simulink model "Switching_06"  (R2022b)
settings: Solver=ode4  StartTime=0.0  StopTime=50  FixedStep=1e-3  MaxStep=1e-3  RelTol=1e-3
undefined symbols (not defined in the file or in its folder): p1, p2, p3, PR_k1, PR_k2, PR_k3, SF_b, SF_xi1, theta_d, tolerance_posture, v_sat, w_sat, x_d, y_d
libraries: simulink x18, dspsigops x6
settings Model: Creator=david  LastModifiedBy=david

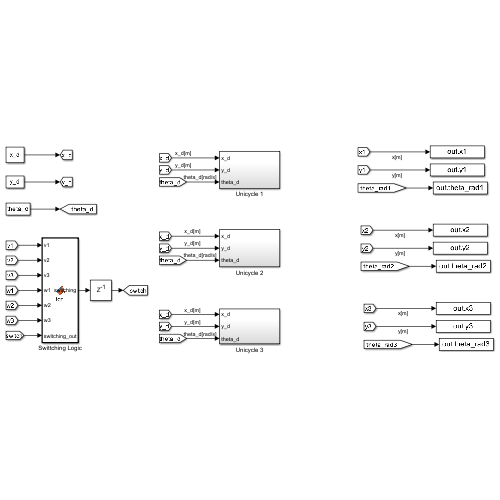
[thumbnail: Simulink's stored preview of the top-level diagram]
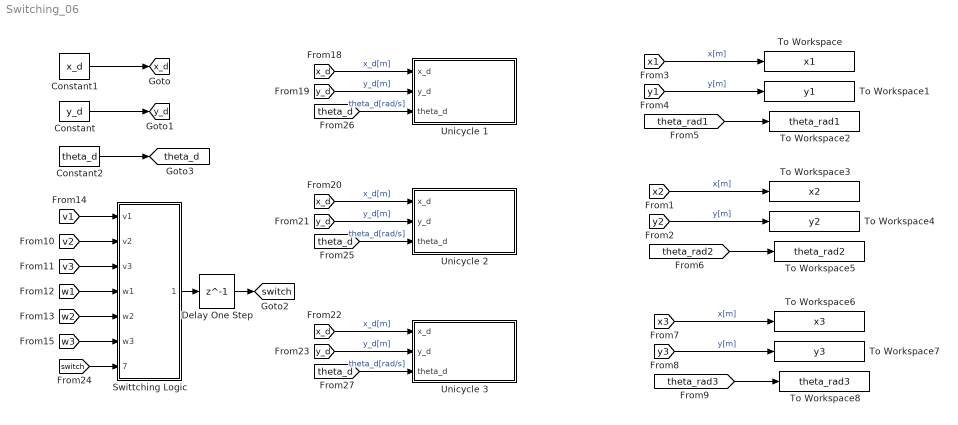
== system Switching_06 ==
  Constant : Constant  Value=y_d
  Constant1 : Constant  Value=x_d
  Constant2 : Constant  Value=theta_d
  Delay One Step : Delay  DelayLength=1
  Swittching Logic : MATLAB Function  TreatAsAtomicUnit=on
  To Workspace : ToWorkspace  VariableName=x1  SaveFormat=Structure With Time  SampleTime=-1
  To Workspace1 : ToWorkspace  VariableName=y1  SaveFormat=Structure With Time  SampleTime=-1
  To Workspace2 : ToWorkspace  VariableName=theta_rad1  SaveFormat=Structure With Time  SampleTime=-1
  To Workspace3 : ToWorkspace  VariableName=x2  SaveFormat=Structure With Time  SampleTime=-1
  To Workspace4 : ToWorkspace  VariableName=y2  SaveFormat=Structure With Time  SampleTime=-1
  To Workspace5 : ToWorkspace  VariableName=theta_rad2  SaveFormat=Structure With Time  SampleTime=-1
  To Workspace6 : ToWorkspace  VariableName=x3  SaveFormat=Structure With Time  SampleTime=-1
  To Workspace7 : ToWorkspace  VariableName=y3  SaveFormat=Structure With Time  SampleTime=-1
  To Workspace8 : ToWorkspace  VariableName=theta_rad3  SaveFormat=Structure With Time  SampleTime=-1
  Unicycle 1 : Subsystem
  Unicycle 2 : Subsystem
  Unicycle 3 : Subsystem
  tag scope: switch=global, theta_d=global, x_d=global, y_d=global
  wires:
  [x1] -> To Workspace/1  "x[m]"
  [y1] -> To Workspace1/1  "y[m]"
  [theta_rad1] -> To Workspace2/1
  [x2] -> To Workspace3/1  "x[m]"
  [y2] -> To Workspace4/1  "y[m]"
  [theta_rad2] -> To Workspace5/1
  [theta_rad3] -> To Workspace8/1
  [y3] -> To Workspace7/1  "y[m]"
  [x3] -> To Workspace6/1  "x[m]"
  [w2] -> Swittching Logic/5(w2)
  [v1] -> Swittching Logic/1(v1)
  [v2] -> Swittching Logic/2(v2)
  Constant2/1 -> [theta_d]
  [w1] -> Swittching Logic/4(w1)
  [v3] -> Swittching Logic/3(v3)
  [x_d] -> Unicycle 1/1(x_d)  "x_d[m]"
  [y_d] -> Unicycle 3/2(y_d)  "y_d[m]"
  [switch] -> Swittching Logic/7(switching_out)
  Swittching Logic/1(switching) -> Delay One Step/1
  [theta_d] -> Unicycle 3/3(theta_d)  "theta_d[rad/s]"
  [x_d] -> Unicycle 2/1(x_d)  "x_d[m]"
  [w3] -> Swittching Logic/6(w3)
  Constant/1 -> [y_d]
  Delay One Step/1 -> [switch]
  [y_d] -> Unicycle 1/2(y_d)  "y_d[m]"
  [theta_d] -> Unicycle 2/3(theta_d)  "theta_d[rad/s]"
  [y_d] -> Unicycle 2/2(y_d)  "y_d[m]"
  [x_d] -> Unicycle 3/1(x_d)  "x_d[m]"
  Constant1/1 -> [x_d]
  [theta_d] -> Unicycle 1/3(theta_d)  "theta_d[rad/s]"

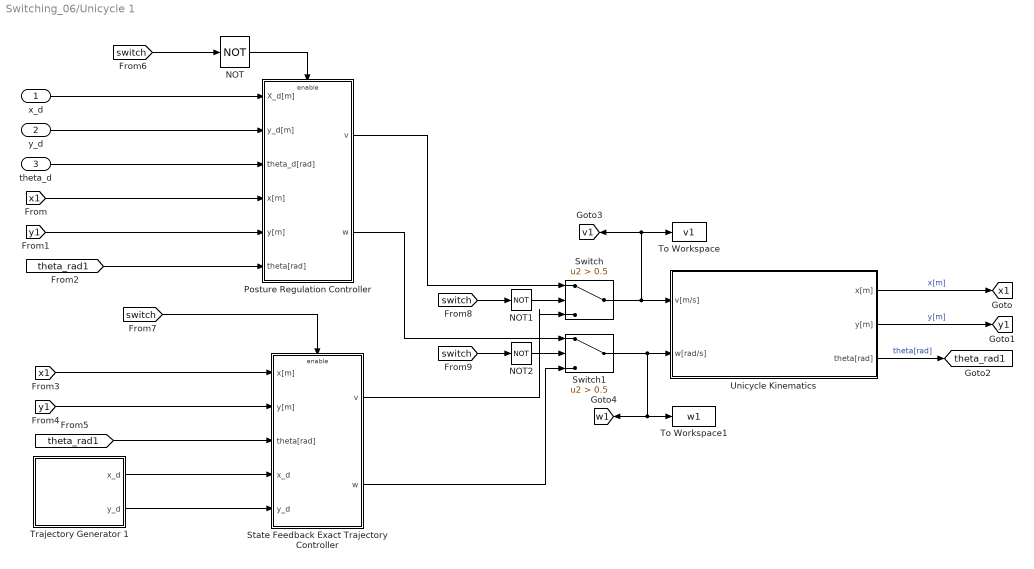
== system Switching_06/Unicycle 1 ==
  x_d : Inport
  y_d : Inport  Port=2
  theta_d : Inport  Port=3
  NOT : Logic  Operator=NOT  IconShape=distinctive  AllPortsSameDT=off  OutDataTypeStr=boolean
  NOT1 : Logic  Operator=NOT  IconShape=distinctive  AllPortsSameDT=off  OutDataTypeStr=boolean
  NOT2 : Logic  Operator=NOT  IconShape=distinctive  AllPortsSameDT=off  OutDataTypeStr=boolean
  Posture Regulation Controller : Subsystem
  State Feedback Exact Trajectory Controller : Subsystem
  Switch : Switch  Criteria=u2 > Threshold  Threshold=0.5  SaturateOnIntegerOverflow=off  InputSameDT=off
  Switch1 : Switch  Criteria=u2 > Threshold  Threshold=0.5  SaturateOnIntegerOverflow=off  InputSameDT=off
  To Workspace : ToWorkspace  VariableName=v1  SaveFormat=Structure With Time  SampleTime=-1
  To Workspace1 : ToWorkspace  VariableName=w1  SaveFormat=Structure With Time  SampleTime=-1
  "Trajectory Generator 1 " : Subsystem
  Unicycle Kinematics : Subsystem
  tag scope: theta_rad1=global, v1=global, w1=global, x1=global, y1=global
  wires:
  Unicycle Kinematics/3(theta[rad]) -> [theta_rad1]  "theta[rad]"
  Unicycle Kinematics/2(y[m]) -> [y1]  "y[m]"
  Unicycle Kinematics/1(x[m]) -> [x1]  "x[m]"
  [theta_rad1] -> State Feedback Exact Trajectory Controller/3(theta[rad])
  [x1] -> State Feedback Exact Trajectory Controller/1(x[m])
  [y1] -> State Feedback Exact Trajectory Controller/2(y[m])
  "Trajectory Generator 1 "/1(x_d) -> State Feedback Exact Trajectory Controller/4(x_d)
  "Trajectory Generator 1 "/2(y_d) -> State Feedback Exact Trajectory Controller/5(y_d)
  [switch] -> State Feedback Exact Trajectory Controller/Enable
  Posture Regulation Controller/2(w) -> Switch1/1
  Posture Regulation Controller/1(v) -> Switch/1
  State Feedback Exact Trajectory Controller/2(w) -> Switch1/3
  [switch] -> NOT2/1
  State Feedback Exact Trajectory Controller/1(v) -> Switch/3
  [switch] -> NOT1/1
  NOT1/1 -> Switch/2
  NOT2/1 -> Switch1/2
  Switch/1 -> Unicycle Kinematics/1(v[m/s]), [v1], To Workspace/1
  Switch1/1 -> Unicycle Kinematics/2(w[rad/s]), To Workspace1/1, [w1]
  [x1] -> Posture Regulation Controller/4(x[m])
  [switch] -> NOT/1
  x_d/1 -> Posture Regulation Controller/1(X_d[m])
  [theta_rad1] -> Posture Regulation Controller/6(theta[rad])
  [y1] -> Posture Regulation Controller/5(y[m])
  y_d/1 -> Posture Regulation Controller/2(y_d[m])
  NOT/1 -> Posture Regulation Controller/Enable
  theta_d/1 -> Posture Regulation Controller/3(theta_d[rad])

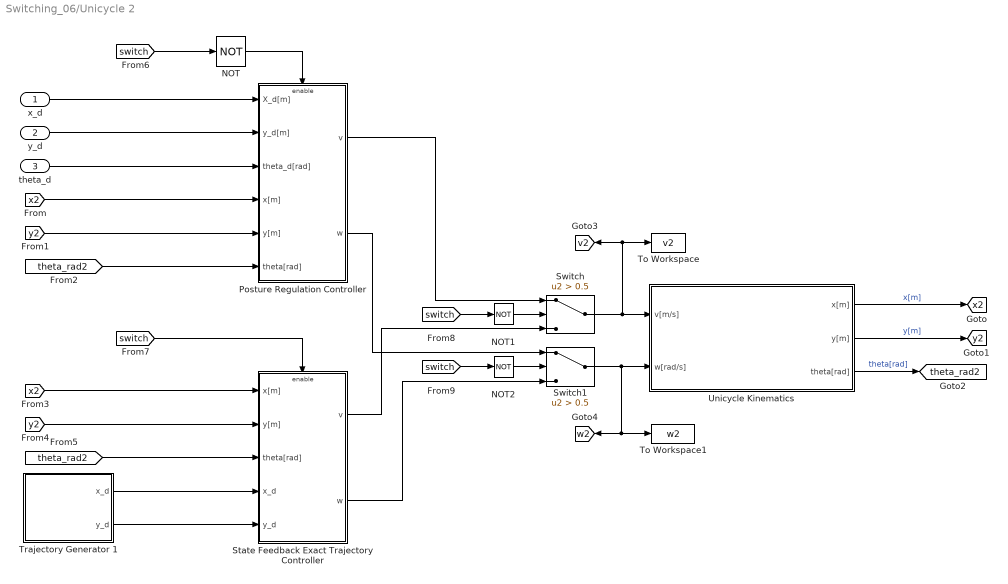
== system Switching_06/Unicycle 2 ==
  x_d : Inport
  y_d : Inport  Port=2
  theta_d : Inport  Port=3
  NOT : Logic  Operator=NOT  IconShape=distinctive  AllPortsSameDT=off  OutDataTypeStr=boolean
  NOT1 : Logic  Operator=NOT  IconShape=distinctive  AllPortsSameDT=off  OutDataTypeStr=boolean
  NOT2 : Logic  Operator=NOT  IconShape=distinctive  AllPortsSameDT=off  OutDataTypeStr=boolean
  Posture Regulation Controller : Subsystem
  State Feedback Exact Trajectory Controller : Subsystem
  Switch : Switch  Criteria=u2 > Threshold  Threshold=0.5  SaturateOnIntegerOverflow=off  InputSameDT=off
  Switch1 : Switch  Criteria=u2 > Threshold  Threshold=0.5  SaturateOnIntegerOverflow=off  InputSameDT=off
  To Workspace : ToWorkspace  VariableName=v2  SaveFormat=Structure With Time  SampleTime=-1
  To Workspace1 : ToWorkspace  VariableName=w2  SaveFormat=Structure With Time  SampleTime=-1
  "Trajectory Generator 1 " : Subsystem
  Unicycle Kinematics : Subsystem
  tag scope: theta_rad2=global, v2=global, w2=global, x2=global, y2=global
  wires:
  Unicycle Kinematics/3(theta[rad]) -> [theta_rad2]  "theta[rad]"
  Unicycle Kinematics/2(y[m]) -> [y2]  "y[m]"
  Unicycle Kinematics/1(x[m]) -> [x2]  "x[m]"
  [switch] -> State Feedback Exact Trajectory Controller/Enable
  Posture Regulation Controller/2(w) -> Switch1/1
  Posture Regulation Controller/1(v) -> Switch/1
  State Feedback Exact Trajectory Controller/2(w) -> Switch1/3
  [switch] -> NOT2/1
  Switch1/1 -> [w2], To Workspace1/1, Unicycle Kinematics/2(w[rad/s])
  [switch] -> NOT1/1
  NOT1/1 -> Switch/2
  NOT2/1 -> Switch1/2
  State Feedback Exact Trajectory Controller/1(v) -> Switch/3
  [theta_rad2] -> State Feedback Exact Trajectory Controller/3(theta[rad])
  [x2] -> State Feedback Exact Trajectory Controller/1(x[m])
  [y2] -> State Feedback Exact Trajectory Controller/2(y[m])
  "Trajectory Generator 1 "/1(x_d) -> State Feedback Exact Trajectory Controller/4(x_d)
  "Trajectory Generator 1 "/2(y_d) -> State Feedback Exact Trajectory Controller/5(y_d)
  theta_d/1 -> Posture Regulation Controller/3(theta_d[rad])
  x_d/1 -> Posture Regulation Controller/1(X_d[m])
  [switch] -> NOT/1
  [x2] -> Posture Regulation Controller/4(x[m])
  [y2] -> Posture Regulation Controller/5(y[m])
  NOT/1 -> Posture Regulation Controller/Enable
  y_d/1 -> Posture Regulation Controller/2(y_d[m])
  [theta_rad2] -> Posture Regulation Controller/6(theta[rad])
  Switch/1 -> To Workspace/1, [v2], Unicycle Kinematics/1(v[m/s])

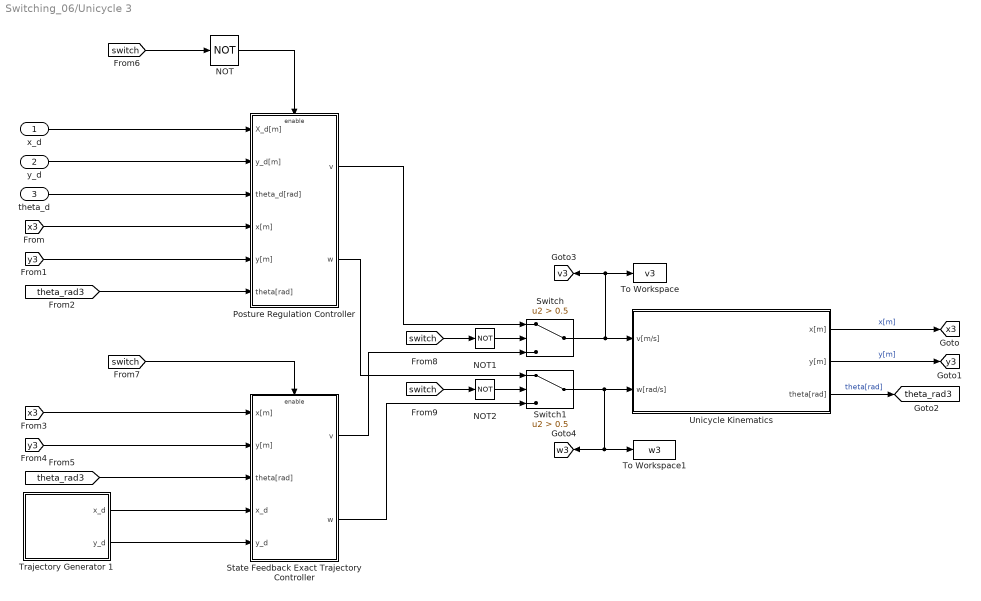
== system Switching_06/Unicycle 3 ==
  x_d : Inport
  y_d : Inport  Port=2
  theta_d : Inport  Port=3
  NOT : Logic  Operator=NOT  IconShape=distinctive  AllPortsSameDT=off  OutDataTypeStr=boolean
  NOT1 : Logic  Operator=NOT  IconShape=distinctive  AllPortsSameDT=off  OutDataTypeStr=boolean
  NOT2 : Logic  Operator=NOT  IconShape=distinctive  AllPortsSameDT=off  OutDataTypeStr=boolean
  Posture Regulation Controller : Subsystem
  State Feedback Exact Trajectory Controller : Subsystem
  Switch : Switch  Criteria=u2 > Threshold  Threshold=0.5  SaturateOnIntegerOverflow=off  InputSameDT=off
  Switch1 : Switch  Criteria=u2 > Threshold  Threshold=0.5  SaturateOnIntegerOverflow=off  InputSameDT=off
  To Workspace : ToWorkspace  VariableName=v3  SaveFormat=Structure With Time  SampleTime=-1
  To Workspace1 : ToWorkspace  VariableName=w3  SaveFormat=Structure With Time  SampleTime=-1
  "Trajectory Generator 1 " : Subsystem
  Unicycle Kinematics : Subsystem
  tag scope: theta_rad3=global, v3=global, w3=global, x3=global, y3=global
  wires:
  Unicycle Kinematics/3(theta[rad]) -> [theta_rad3]  "theta[rad]"
  Unicycle Kinematics/2(y[m]) -> [y3]  "y[m]"
  Unicycle Kinematics/1(x[m]) -> [x3]  "x[m]"
  [switch] -> State Feedback Exact Trajectory Controller/Enable
  Posture Regulation Controller/1(v) -> Switch/1
  [switch] -> NOT1/1
  [switch] -> NOT2/1
  Posture Regulation Controller/2(w) -> Switch1/1
  NOT1/1 -> Switch/2
  NOT2/1 -> Switch1/2
  [theta_rad3] -> State Feedback Exact Trajectory Controller/3(theta[rad])
  [x3] -> State Feedback Exact Trajectory Controller/1(x[m])
  [y3] -> State Feedback Exact Trajectory Controller/2(y[m])
  "Trajectory Generator 1 "/1(x_d) -> State Feedback Exact Trajectory Controller/4(x_d)
  "Trajectory Generator 1 "/2(y_d) -> State Feedback Exact Trajectory Controller/5(y_d)
  State Feedback Exact Trajectory Controller/1(v) -> Switch/3
  State Feedback Exact Trajectory Controller/2(w) -> Switch1/3
  Switch/1 -> Unicycle Kinematics/1(v[m/s]), To Workspace/1, [v3]
  Switch1/1 -> [w3], To Workspace1/1, Unicycle Kinematics/2(w[rad/s])
  y_d/1 -> Posture Regulation Controller/2(y_d[m])
  [y3] -> Posture Regulation Controller/5(y[m])
  [x3] -> Posture Regulation Controller/4(x[m])
  x_d/1 -> Posture Regulation Controller/1(X_d[m])
  theta_d/1 -> Posture Regulation Controller/3(theta_d[rad])
  [switch] -> NOT/1
  NOT/1 -> Posture Regulation Controller/Enable
  [theta_rad3] -> Posture Regulation Controller/6(theta[rad])

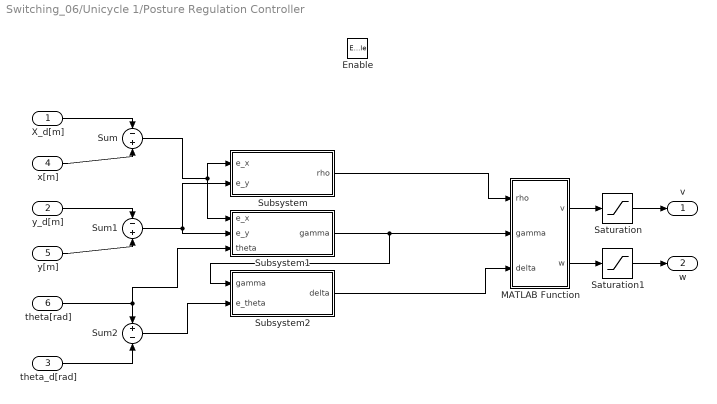
== system Switching_06/Unicycle 1/Posture Regulation Controller ==
  X_d[m] : Inport
  y_d[m] : Inport  Port=2
  theta_d[rad] : Inport  Port=3
  x[m] : Inport  Port=4
  y[m] : Inport  Port=5
  theta[rad] : Inport  Port=6
  Enable : EnablePort
  MATLAB Function : MATLAB Function  TreatAsAtomicUnit=on
  Saturation : Saturate  UpperLimit=v_sat  LowerLimit=-v_sat
  Saturation1 : Saturate  UpperLimit=w_sat  LowerLimit=-w_sat
  Subsystem : Subsystem
  Subsystem1 : Subsystem
  Subsystem2 : Subsystem
  Sum : Sum  Inputs=-+
  Sum1 : Sum  Inputs=-+
  Sum2 : Sum  Inputs=+-
  v : Outport
  w : Outport  Port=2
  wires:
  X_d[m]/1 -> Sum/1
  x[m]/1 -> Sum/2
  y_d[m]/1 -> Sum1/1
  y[m]/1 -> Sum1/2
  Sum1/1 -> Subsystem1/2(e_y), Subsystem/2(e_y)
  Sum2/1 -> Subsystem2/2(e_theta)
  Subsystem1/1(gamma) -> MATLAB Function/2(gamma), Subsystem2/1(gamma)
  Subsystem2/1(delta) -> MATLAB Function/3(delta)
  Subsystem/1(rho) -> MATLAB Function/1(rho)
  Sum/1 -> Subsystem1/1(e_x), Subsystem/1(e_x)
  MATLAB Function/1(v) -> Saturation/1
  MATLAB Function/2(w) -> Saturation1/1
  theta[rad]/1 -> Sum2/1, Subsystem1/3(theta)
  theta_d[rad]/1 -> Sum2/2
  Saturation/1 -> v/1
  Saturation1/1 -> w/1

== system Switching_06/Unicycle 1/State Feedback Exact Trajectory Controller ==
  x[m] : Inport
  y[m] : Inport  Port=2
  theta[rad] : Inport  Port=3
  x_d : Inport  Port=4
  y_d : Inport  Port=5
  Enable : EnablePort
  Controller : Subsystem
  Differential Flatness : Subsystem
  v : Outport
  w : Outport  Port=2
  wires:
  Controller/2(w) -> w/1
  Controller/1(v) -> v/1
  Differential Flatness/3(w_d) -> Controller/3(w_d)
  Differential Flatness/1(q_d) -> Controller/1(q_d)
  Differential Flatness/2(v_d) -> Controller/2(v_d)
  y_d/1 -> Differential Flatness/2(y_d)
  x_d/1 -> Differential Flatness/1(x_d)
  x[m]/1 -> Controller/4(x)
  y[m]/1 -> Controller/5(y)
  theta[rad]/1 -> Controller/6(theta)

== system Switching_06/Unicycle 1/Trajectory Generator 1  ==
  Repeating Sequence : simulink/Sources/Repeating Sequence  rep_seq_t=time  rep_seq_y=y_d1
  Repeating Sequence1 : simulink/Sources/Repeating Sequence  rep_seq_t=time  rep_seq_y=x_d1
  To Workspace2 : ToWorkspace  VariableName=y_d1  SaveFormat=Structure With Time  SampleTime=-1
  To Workspace3 : ToWorkspace  VariableName=x_d1  SaveFormat=Structure With Time  SampleTime=-1
  x_d : Outport
  y_d : Outport  Port=2
  wires:
  Repeating Sequence1/1 -> x_d/1, To Workspace3/1
  Repeating Sequence/1 -> To Workspace2/1, y_d/1

== system Switching_06/Unicycle 1/Unicycle Kinematics ==
  v[m/s] : Inport
  w[rad/s] : Inport  Port=2
  Cos : Trigonometry  Operator=cos
  Cos1 : Trigonometry
  Integrator : Integrator  InitialCondition=p1(1)
  Integrator1 : Integrator  InitialCondition=p1(2)
  Integrator2 : Integrator  InitialCondition=p1(3)
  Product : Product
  Product1 : Product
  x[m] : Outport
  y[m] : Outport  Port=2
  theta[rad] : Outport  Port=3
  wires:
  Integrator/1 -> x[m]/1  "x"
  Integrator1/1 -> y[m]/1  "y"
  w[rad/s]/1 -> Integrator2/1  "theta_dot"
  Integrator2/1 -> Cos/1, Cos1/1, theta[rad]/1  "theta[rad]"
  Product/1 -> Integrator/1  "x_dot"
  Cos1/1 -> Product1/2
  Cos/1 -> Product/1
  v[m/s]/1 -> Product1/1, Product/2
  Product1/1 -> Integrator1/1  "y_dot"

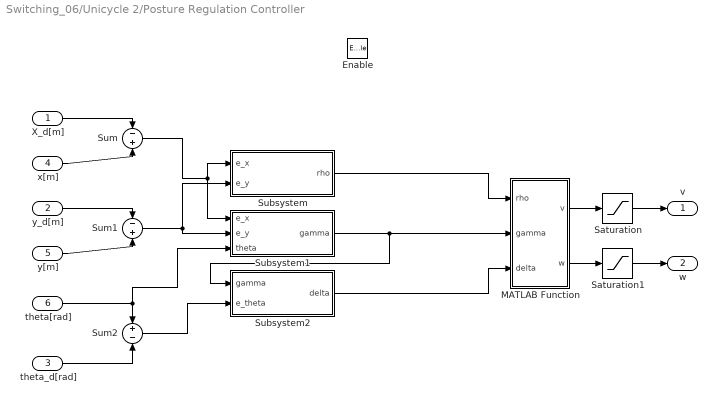
== system Switching_06/Unicycle 2/Posture Regulation Controller ==
  X_d[m] : Inport
  y_d[m] : Inport  Port=2
  theta_d[rad] : Inport  Port=3
  x[m] : Inport  Port=4
  y[m] : Inport  Port=5
  theta[rad] : Inport  Port=6
  Enable : EnablePort
  MATLAB Function : MATLAB Function  TreatAsAtomicUnit=on
  Saturation : Saturate  UpperLimit=v_sat  LowerLimit=-v_sat
  Saturation1 : Saturate  UpperLimit=w_sat  LowerLimit=-w_sat
  Subsystem : Subsystem
  Subsystem1 : Subsystem
  Subsystem2 : Subsystem
  Sum : Sum  Inputs=-+
  Sum1 : Sum  Inputs=-+
  Sum2 : Sum  Inputs=+-
  v : Outport
  w : Outport  Port=2
  wires:
  X_d[m]/1 -> Sum/1
  x[m]/1 -> Sum/2
  y_d[m]/1 -> Sum1/1
  y[m]/1 -> Sum1/2
  Sum1/1 -> Subsystem1/2(e_y), Subsystem/2(e_y)
  Sum2/1 -> Subsystem2/2(e_theta)
  Subsystem1/1(gamma) -> MATLAB Function/2(gamma), Subsystem2/1(gamma)
  Subsystem2/1(delta) -> MATLAB Function/3(delta)
  Subsystem/1(rho) -> MATLAB Function/1(rho)
  Sum/1 -> Subsystem1/1(e_x), Subsystem/1(e_x)
  MATLAB Function/1(v) -> Saturation/1
  MATLAB Function/2(w) -> Saturation1/1
  theta[rad]/1 -> Sum2/1, Subsystem1/3(theta)
  theta_d[rad]/1 -> Sum2/2
  Saturation/1 -> v/1
  Saturation1/1 -> w/1

== system Switching_06/Unicycle 2/State Feedback Exact Trajectory Controller ==
  x[m] : Inport
  y[m] : Inport  Port=2
  theta[rad] : Inport  Port=3
  x_d : Inport  Port=4
  y_d : Inport  Port=5
  Enable : EnablePort
  Controller : Subsystem
  Differential Flatness : Subsystem
  v : Outport
  w : Outport  Port=2
  wires:
  Controller/2(w) -> w/1
  Controller/1(v) -> v/1
  Differential Flatness/3(w_d) -> Controller/3(w_d)
  Differential Flatness/1(q_d) -> Controller/1(q_d)
  Differential Flatness/2(v_d) -> Controller/2(v_d)
  y_d/1 -> Differential Flatness/2(y_d)
  x_d/1 -> Differential Flatness/1(x_d)
  x[m]/1 -> Controller/4(x)
  y[m]/1 -> Controller/5(y)
  theta[rad]/1 -> Controller/6(theta)

== system Switching_06/Unicycle 2/Trajectory Generator 1  ==
  Repeating Sequence : simulink/Sources/Repeating Sequence  rep_seq_t=time  rep_seq_y=y_d2
  Repeating Sequence1 : simulink/Sources/Repeating Sequence  rep_seq_t=time  rep_seq_y=x_d2
  To Workspace2 : ToWorkspace  VariableName=y_d2  SaveFormat=Structure With Time  SampleTime=-1
  To Workspace3 : ToWorkspace  VariableName=x_d2  SaveFormat=Structure With Time  SampleTime=-1
  x_d : Outport
  y_d : Outport  Port=2
  wires:
  Repeating Sequence1/1 -> x_d/1, To Workspace3/1
  Repeating Sequence/1 -> To Workspace2/1, y_d/1

== system Switching_06/Unicycle 2/Unicycle Kinematics ==
  v[m/s] : Inport
  w[rad/s] : Inport  Port=2
  Cos : Trigonometry  Operator=cos
  Cos1 : Trigonometry
  Integrator : Integrator  InitialCondition=p2(1)
  Integrator1 : Integrator  InitialCondition=p2(2)
  Integrator2 : Integrator  InitialCondition=p2(3)
  Product : Product
  Product1 : Product
  x[m] : Outport
  y[m] : Outport  Port=2
  theta[rad] : Outport  Port=3
  wires:
  Integrator/1 -> x[m]/1  "x"
  Integrator1/1 -> y[m]/1  "y"
  w[rad/s]/1 -> Integrator2/1  "theta_dot"
  Integrator2/1 -> Cos/1, Cos1/1, theta[rad]/1  "theta[rad]"
  Product/1 -> Integrator/1  "x_dot"
  Cos1/1 -> Product1/2
  Cos/1 -> Product/1
  v[m/s]/1 -> Product1/1, Product/2
  Product1/1 -> Integrator1/1  "y_dot"

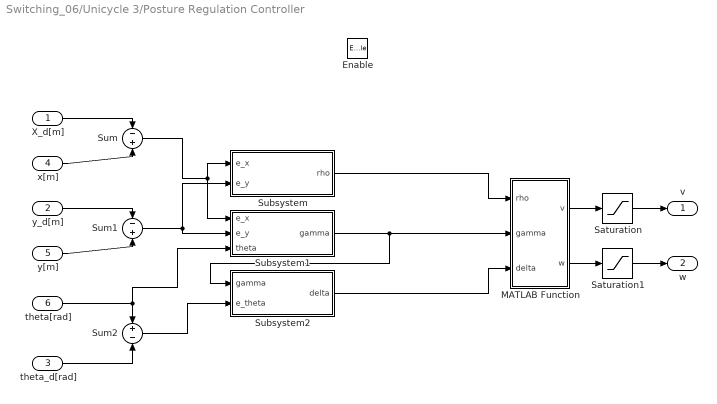
== system Switching_06/Unicycle 3/Posture Regulation Controller ==
  X_d[m] : Inport
  y_d[m] : Inport  Port=2
  theta_d[rad] : Inport  Port=3
  x[m] : Inport  Port=4
  y[m] : Inport  Port=5
  theta[rad] : Inport  Port=6
  Enable : EnablePort
  MATLAB Function : MATLAB Function  TreatAsAtomicUnit=on
  Saturation : Saturate  UpperLimit=v_sat  LowerLimit=-v_sat
  Saturation1 : Saturate  UpperLimit=w_sat  LowerLimit=-w_sat
  Subsystem : Subsystem
  Subsystem1 : Subsystem
  Subsystem2 : Subsystem
  Sum : Sum  Inputs=-+
  Sum1 : Sum  Inputs=-+
  Sum2 : Sum  Inputs=+-
  v : Outport
  w : Outport  Port=2
  wires:
  X_d[m]/1 -> Sum/1
  x[m]/1 -> Sum/2
  y_d[m]/1 -> Sum1/1
  y[m]/1 -> Sum1/2
  Sum1/1 -> Subsystem1/2(e_y), Subsystem/2(e_y)
  Sum2/1 -> Subsystem2/2(e_theta)
  Subsystem1/1(gamma) -> MATLAB Function/2(gamma), Subsystem2/1(gamma)
  Subsystem2/1(delta) -> MATLAB Function/3(delta)
  Subsystem/1(rho) -> MATLAB Function/1(rho)
  Sum/1 -> Subsystem1/1(e_x), Subsystem/1(e_x)
  MATLAB Function/1(v) -> Saturation/1
  MATLAB Function/2(w) -> Saturation1/1
  theta[rad]/1 -> Sum2/1, Subsystem1/3(theta)
  theta_d[rad]/1 -> Sum2/2
  Saturation1/1 -> w/1
  Saturation/1 -> v/1

== system Switching_06/Unicycle 3/State Feedback Exact Trajectory Controller ==
  x[m] : Inport
  y[m] : Inport  Port=2
  theta[rad] : Inport  Port=3
  x_d : Inport  Port=4
  y_d : Inport  Port=5
  Enable : EnablePort
  Controller : Subsystem
  Differential Flatness : Subsystem
  v : Outport
  w : Outport  Port=2
  wires:
  Controller/2(w) -> w/1
  Controller/1(v) -> v/1
  Differential Flatness/3(w_d) -> Controller/3(w_d)
  Differential Flatness/1(q_d) -> Controller/1(q_d)
  Differential Flatness/2(v_d) -> Controller/2(v_d)
  y_d/1 -> Differential Flatness/2(y_d)
  x_d/1 -> Differential Flatness/1(x_d)
  x[m]/1 -> Controller/4(x)
  y[m]/1 -> Controller/5(y)
  theta[rad]/1 -> Controller/6(theta)

== system Switching_06/Unicycle 3/Trajectory Generator 1  ==
  Repeating Sequence : simulink/Sources/Repeating Sequence  rep_seq_t=time  rep_seq_y=y_d3
  Repeating Sequence1 : simulink/Sources/Repeating Sequence  rep_seq_t=time  rep_seq_y=x_d3
  To Workspace2 : ToWorkspace  VariableName=y_d3  SaveFormat=Structure With Time  SampleTime=-1
  To Workspace3 : ToWorkspace  VariableName=x_d3  SaveFormat=Structure With Time  SampleTime=-1
  x_d : Outport
  y_d : Outport  Port=2
  wires:
  Repeating Sequence1/1 -> x_d/1, To Workspace3/1
  Repeating Sequence/1 -> y_d/1, To Workspace2/1

== system Switching_06/Unicycle 3/Unicycle Kinematics ==
  v[m/s] : Inport
  w[rad/s] : Inport  Port=2
  Cos : Trigonometry  Operator=cos
  Cos1 : Trigonometry
  Integrator : Integrator  InitialCondition=p3(1)
  Integrator1 : Integrator  InitialCondition=p3(2)
  Integrator2 : Integrator  InitialCondition=p3(3)
  Product : Product
  Product1 : Product
  x[m] : Outport
  y[m] : Outport  Port=2
  theta[rad] : Outport  Port=3
  wires:
  Integrator/1 -> x[m]/1  "x"
  Integrator1/1 -> y[m]/1  "y"
  w[rad/s]/1 -> Integrator2/1  "theta_dot"
  Integrator2/1 -> Cos/1, Cos1/1, theta[rad]/1  "theta[rad]"
  Product/1 -> Integrator/1  "x_dot"
  Cos1/1 -> Product1/2
  Cos/1 -> Product/1
  v[m/s]/1 -> Product1/1, Product/2
  Product1/1 -> Integrator1/1  "y_dot"

== system Switching_06/Unicycle 1/Posture Regulation Controller/Subsystem ==
  e_x : Inport
  e_y : Inport  Port=2
  Sqrt : Sqrt
  Square : Math  Operator=square
  Square1 : Math  Operator=square
  Sum : Sum
  rho : Outport
  wires:
  Sqrt/1 -> rho/1
  e_x/1 -> Square/1
  e_y/1 -> Square1/1
  Sum/1 -> Sqrt/1
  Square/1 -> Sum/1
  Square1/1 -> Sum/2

== system Switching_06/Unicycle 1/Posture Regulation Controller/Subsystem1 ==
  e_x : Inport
  e_y : Inport  Port=2
  theta : Inport  Port=3
  Atan2 : Trigonometry  Operator=atan2
  Constant : Constant  Value=pi
  Sum : Sum  Inputs=+-+
  Unwrap : dspsigops/Unwrap  tol=pi  InputProcessing=Columns as channels (frame based)  running=off
  gamma : Outport
  wires:
  e_x/1 -> Atan2/2
  e_y/1 -> Atan2/1
  theta/1 -> Sum/2
  Sum/1 -> gamma/1
  Atan2/1 -> Unwrap/1
  Constant/1 -> Sum/3
  Unwrap/1 -> Sum/1

== system Switching_06/Unicycle 1/Posture Regulation Controller/Subsystem2 ==
  gamma : Inport
  e_theta : Inport  Port=2
  Sum : Sum
  delta : Outport
  wires:
  e_theta/1 -> Sum/2
  Sum/1 -> delta/1
  gamma/1 -> Sum/1

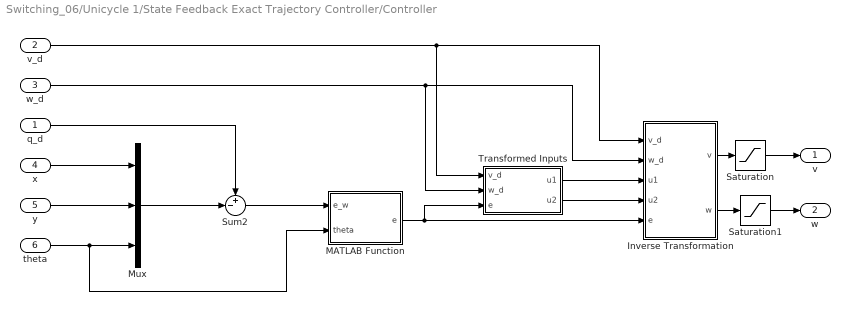
== system Switching_06/Unicycle 1/State Feedback Exact Trajectory Controller/Controller ==
  q_d : Inport
  v_d : Inport  Port=2
  w_d : Inport  Port=3
  x : Inport  Port=4
  y : Inport  Port=5
  theta : Inport  Port=6
  Inverse Transformation : MATLAB Function  TreatAsAtomicUnit=on
  MATLAB Function : MATLAB Function  TreatAsAtomicUnit=on
  Mux : Mux  Inputs=3
  Saturation : Saturate  UpperLimit=v_sat  LowerLimit=-v_sat
  Saturation1 : Saturate  UpperLimit=w_sat  LowerLimit=-w_sat
  Sum2 : Sum  Inputs=+-|
  Transformed Inputs : MATLAB Function  TreatAsAtomicUnit=on
  v : Outport
  w : Outport  Port=2
  wires:
  q_d/1 -> Sum2/1
  MATLAB Function/1(e) -> Inverse Transformation/5(e), Transformed Inputs/3(e)
  Transformed Inputs/1(u1) -> Inverse Transformation/3(u1)
  Transformed Inputs/2(u2) -> Inverse Transformation/4(u2)
  Inverse Transformation/1(v) -> Saturation/1
  Inverse Transformation/2(w) -> Saturation1/1
  x/1 -> Mux/1
  y/1 -> Mux/2
  theta/1 -> Mux/3, MATLAB Function/2(theta)
  Mux/1 -> Sum2/2
  Sum2/1 -> MATLAB Function/1(e_w)
  w_d/1 -> Inverse Transformation/2(w_d), Transformed Inputs/2(w_d)
  v_d/1 -> Transformed Inputs/1(v_d), Inverse Transformation/1(v_d)
  Saturation/1 -> v/1
  Saturation1/1 -> w/1

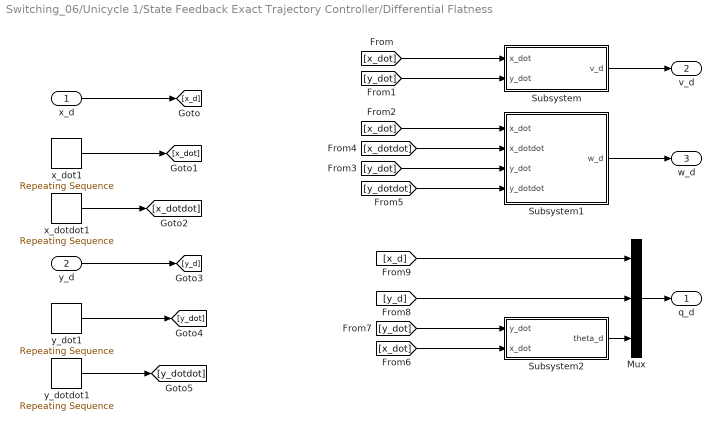
== system Switching_06/Unicycle 1/State Feedback Exact Trajectory Controller/Differential Flatness ==
  x_d : Inport
  y_d : Inport  Port=2
  Mux : Mux  Inputs=3
  Subsystem : Subsystem
  Subsystem1 : Subsystem
  Subsystem2 : Subsystem
  x_dot1 : simulink/Sources/Repeating Sequence  rep_seq_t=time  rep_seq_y=x_dot1
  x_dotdot1 : simulink/Sources/Repeating Sequence  rep_seq_t=time  rep_seq_y=x_dotdot1
  y_dot1 : simulink/Sources/Repeating Sequence  rep_seq_t=time  rep_seq_y=y_dot1
  y_dotdot1 : simulink/Sources/Repeating Sequence  rep_seq_t=time  rep_seq_y=y_dotdot1
  q_d : Outport
  v_d : Outport  Port=2
  w_d : Outport  Port=3
  wires:
  Subsystem/1(v_d) -> v_d/1
  [x_dot] -> Subsystem/1(x_dot)
  [y_dot] -> Subsystem/2(y_dot)
  [x_dot] -> Subsystem1/1(x_dot)
  [x_dotdot] -> Subsystem1/2(x_dotdot)
  Subsystem1/1(w_d) -> w_d/1
  [y_dot] -> Subsystem1/3(y_dot)
  [y_dotdot] -> Subsystem1/4(y_dotdot)
  Subsystem2/1(theta_d) -> Mux/3
  [y_d] -> Mux/2
  [x_d] -> Mux/1
  Mux/1 -> q_d/1
  [y_dot] -> Subsystem2/1(y_dot)
  [x_dot] -> Subsystem2/2(x_dot)
  y_d/1 -> [y_d]
  y_dotdot1/1 -> [y_dotdot]
  x_dot1/1 -> [x_dot]
  x_d/1 -> [x_d]
  y_dot1/1 -> [y_dot]
  x_dotdot1/1 -> [x_dotdot]

== system Switching_06/Unicycle 2/Posture Regulation Controller/Subsystem ==
  e_x : Inport
  e_y : Inport  Port=2
  Sqrt : Sqrt
  Square : Math  Operator=square
  Square1 : Math  Operator=square
  Sum : Sum
  rho : Outport
  wires:
  Sqrt/1 -> rho/1
  e_x/1 -> Square/1
  e_y/1 -> Square1/1
  Sum/1 -> Sqrt/1
  Square/1 -> Sum/1
  Square1/1 -> Sum/2

== system Switching_06/Unicycle 2/Posture Regulation Controller/Subsystem1 ==
  e_x : Inport
  e_y : Inport  Port=2
  theta : Inport  Port=3
  Atan2 : Trigonometry  Operator=atan2
  Constant : Constant  Value=pi
  Sum : Sum  Inputs=+-+
  Unwrap : dspsigops/Unwrap  tol=pi  InputProcessing=Columns as channels (frame based)  running=off
  gamma : Outport
  wires:
  e_x/1 -> Atan2/2
  e_y/1 -> Atan2/1
  theta/1 -> Sum/2
  Sum/1 -> gamma/1
  Atan2/1 -> Unwrap/1
  Constant/1 -> Sum/3
  Unwrap/1 -> Sum/1

== system Switching_06/Unicycle 2/Posture Regulation Controller/Subsystem2 ==
  gamma : Inport
  e_theta : Inport  Port=2
  Sum : Sum
  delta : Outport
  wires:
  e_theta/1 -> Sum/2
  Sum/1 -> delta/1
  gamma/1 -> Sum/1

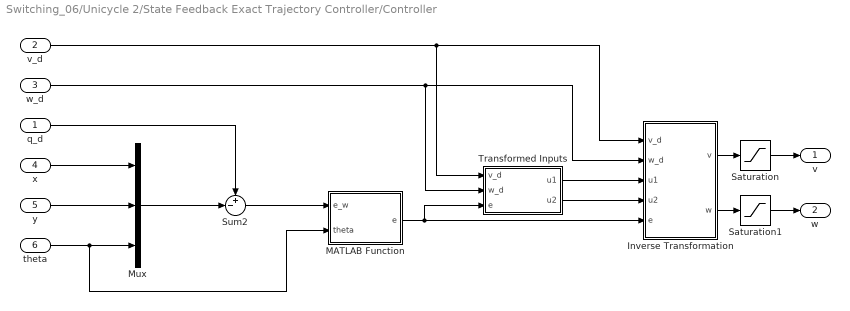
== system Switching_06/Unicycle 2/State Feedback Exact Trajectory Controller/Controller ==
  q_d : Inport
  v_d : Inport  Port=2
  w_d : Inport  Port=3
  x : Inport  Port=4
  y : Inport  Port=5
  theta : Inport  Port=6
  Inverse Transformation : MATLAB Function  TreatAsAtomicUnit=on
  MATLAB Function : MATLAB Function  TreatAsAtomicUnit=on
  Mux : Mux  Inputs=3
  Saturation : Saturate  UpperLimit=v_sat  LowerLimit=-v_sat
  Saturation1 : Saturate  UpperLimit=w_sat  LowerLimit=-w_sat
  Sum2 : Sum  Inputs=+-|
  Transformed Inputs : MATLAB Function  TreatAsAtomicUnit=on
  v : Outport
  w : Outport  Port=2
  wires:
  q_d/1 -> Sum2/1
  MATLAB Function/1(e) -> Inverse Transformation/5(e), Transformed Inputs/3(e)
  Transformed Inputs/1(u1) -> Inverse Transformation/3(u1)
  Transformed Inputs/2(u2) -> Inverse Transformation/4(u2)
  Inverse Transformation/1(v) -> Saturation/1
  Inverse Transformation/2(w) -> Saturation1/1
  x/1 -> Mux/1
  y/1 -> Mux/2
  theta/1 -> Mux/3, MATLAB Function/2(theta)
  Mux/1 -> Sum2/2
  Sum2/1 -> MATLAB Function/1(e_w)
  w_d/1 -> Inverse Transformation/2(w_d), Transformed Inputs/2(w_d)
  v_d/1 -> Transformed Inputs/1(v_d), Inverse Transformation/1(v_d)
  Saturation/1 -> v/1
  Saturation1/1 -> w/1

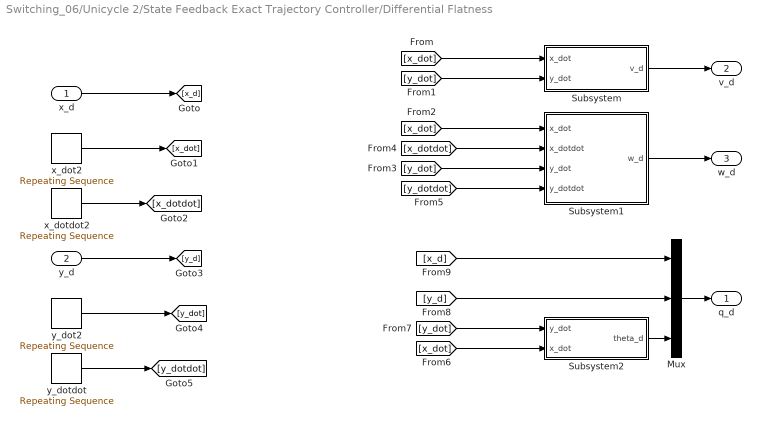
== system Switching_06/Unicycle 2/State Feedback Exact Trajectory Controller/Differential Flatness ==
  x_d : Inport
  y_d : Inport  Port=2
  Mux : Mux  Inputs=3
  Subsystem : Subsystem
  Subsystem1 : Subsystem
  Subsystem2 : Subsystem
  x_dot2 : simulink/Sources/Repeating Sequence  rep_seq_t=time  rep_seq_y=x_dot2
  x_dotdot2 : simulink/Sources/Repeating Sequence  rep_seq_t=time  rep_seq_y=x_dotdot2
  y_dot2 : simulink/Sources/Repeating Sequence  rep_seq_t=time  rep_seq_y=y_dot2
  y_dotdot : simulink/Sources/Repeating Sequence  rep_seq_t=time  rep_seq_y=y_dotdot2
  q_d : Outport
  v_d : Outport  Port=2
  w_d : Outport  Port=3
  wires:
  Subsystem/1(v_d) -> v_d/1
  [x_dot] -> Subsystem/1(x_dot)
  [y_dot] -> Subsystem/2(y_dot)
  [x_dot] -> Subsystem1/1(x_dot)
  [x_dotdot] -> Subsystem1/2(x_dotdot)
  Subsystem1/1(w_d) -> w_d/1
  [y_dot] -> Subsystem1/3(y_dot)
  [y_dotdot] -> Subsystem1/4(y_dotdot)
  Subsystem2/1(theta_d) -> Mux/3
  [y_d] -> Mux/2
  [x_d] -> Mux/1
  Mux/1 -> q_d/1
  [y_dot] -> Subsystem2/1(y_dot)
  [x_dot] -> Subsystem2/2(x_dot)
  y_d/1 -> [y_d]
  x_dotdot2/1 -> [x_dotdot]
  x_d/1 -> [x_d]
  x_dot2/1 -> [x_dot]
  y_dotdot/1 -> [y_dotdot]
  y_dot2/1 -> [y_dot]

== system Switching_06/Unicycle 3/Posture Regulation Controller/Subsystem ==
  e_x : Inport
  e_y : Inport  Port=2
  Sqrt : Sqrt
  Square : Math  Operator=square
  Square1 : Math  Operator=square
  Sum : Sum
  rho : Outport
  wires:
  Sqrt/1 -> rho/1
  e_x/1 -> Square/1
  e_y/1 -> Square1/1
  Sum/1 -> Sqrt/1
  Square/1 -> Sum/1
  Square1/1 -> Sum/2

== system Switching_06/Unicycle 3/Posture Regulation Controller/Subsystem1 ==
  e_x : Inport
  e_y : Inport  Port=2
  theta : Inport  Port=3
  Atan2 : Trigonometry  Operator=atan2
  Constant : Constant  Value=pi
  Sum : Sum  Inputs=+-+
  Unwrap : dspsigops/Unwrap  tol=pi  InputProcessing=Columns as channels (frame based)  running=off
  gamma : Outport
  wires:
  e_x/1 -> Atan2/2
  e_y/1 -> Atan2/1
  theta/1 -> Sum/2
  Sum/1 -> gamma/1
  Atan2/1 -> Unwrap/1
  Constant/1 -> Sum/3
  Unwrap/1 -> Sum/1

== system Switching_06/Unicycle 3/Posture Regulation Controller/Subsystem2 ==
  gamma : Inport
  e_theta : Inport  Port=2
  Sum : Sum
  delta : Outport
  wires:
  e_theta/1 -> Sum/2
  Sum/1 -> delta/1
  gamma/1 -> Sum/1

== system Switching_06/Unicycle 3/State Feedback Exact Trajectory Controller/Controller ==
  q_d : Inport
  v_d : Inport  Port=2
  w_d : Inport  Port=3
  x : Inport  Port=4
  y : Inport  Port=5
  theta : Inport  Port=6
  Inverse Transformation : MATLAB Function  TreatAsAtomicUnit=on
  MATLAB Function : MATLAB Function  TreatAsAtomicUnit=on
  Mux : Mux  Inputs=3
  Saturation : Saturate  UpperLimit=v_sat  LowerLimit=-v_sat
  Saturation1 : Saturate  UpperLimit=w_sat  LowerLimit=-w_sat
  Sum2 : Sum  Inputs=+-|
  Transformed Inputs : MATLAB Function  TreatAsAtomicUnit=on
  v : Outport
  w : Outport  Port=2
  wires:
  q_d/1 -> Sum2/1
  MATLAB Function/1(e) -> Inverse Transformation/5(e), Transformed Inputs/3(e)
  Transformed Inputs/1(u1) -> Inverse Transformation/3(u1)
  Transformed Inputs/2(u2) -> Inverse Transformation/4(u2)
  Inverse Transformation/1(v) -> Saturation/1
  Inverse Transformation/2(w) -> Saturation1/1
  x/1 -> Mux/1
  y/1 -> Mux/2
  theta/1 -> Mux/3, MATLAB Function/2(theta)
  Mux/1 -> Sum2/2
  Sum2/1 -> MATLAB Function/1(e_w)
  w_d/1 -> Inverse Transformation/2(w_d), Transformed Inputs/2(w_d)
  v_d/1 -> Transformed Inputs/1(v_d), Inverse Transformation/1(v_d)
  Saturation/1 -> v/1
  Saturation1/1 -> w/1

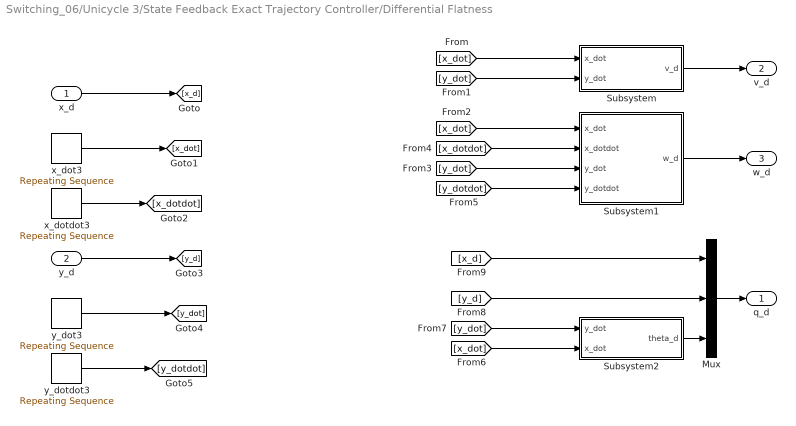
== system Switching_06/Unicycle 3/State Feedback Exact Trajectory Controller/Differential Flatness ==
  x_d : Inport
  y_d : Inport  Port=2
  Mux : Mux  Inputs=3
  Subsystem : Subsystem
  Subsystem1 : Subsystem
  Subsystem2 : Subsystem
  x_dot3 : simulink/Sources/Repeating Sequence  rep_seq_t=time  rep_seq_y=x_dot3
  x_dotdot3 : simulink/Sources/Repeating Sequence  rep_seq_t=time  rep_seq_y=x_dotdot3
  y_dot3 : simulink/Sources/Repeating Sequence  rep_seq_t=time  rep_seq_y=y_dot3
  y_dotdot3 : simulink/Sources/Repeating Sequence  rep_seq_t=time  rep_seq_y=y_dotdot3
  q_d : Outport
  v_d : Outport  Port=2
  w_d : Outport  Port=3
  wires:
  Subsystem/1(v_d) -> v_d/1
  [x_dot] -> Subsystem/1(x_dot)
  [y_dot] -> Subsystem/2(y_dot)
  [x_dot] -> Subsystem1/1(x_dot)
  [x_dotdot] -> Subsystem1/2(x_dotdot)
  Subsystem1/1(w_d) -> w_d/1
  [y_dot] -> Subsystem1/3(y_dot)
  [y_dotdot] -> Subsystem1/4(y_dotdot)
  Subsystem2/1(theta_d) -> Mux/3
  [y_d] -> Mux/2
  [x_d] -> Mux/1
  Mux/1 -> q_d/1
  [y_dot] -> Subsystem2/1(y_dot)
  [x_dot] -> Subsystem2/2(x_dot)
  y_dot3/1 -> [y_dot]
  y_dotdot3/1 -> [y_dotdot]
  x_d/1 -> [x_d]
  y_d/1 -> [y_d]
  x_dotdot3/1 -> [x_dotdot]
  x_dot3/1 -> [x_dot]

== system Switching_06/Unicycle 1/State Feedback Exact Trajectory Controller/Differential Flatness/Subsystem ==
  x_dot : Inport
  y_dot : Inport  Port=2
  Square : Math  Operator=square
  Square Root : Sqrt
  Square1 : Math  Operator=square
  Sum : Sum
  v_d : Outport
  wires:
  x_dot/1 -> Square/1
  y_dot/1 -> Square1/1
  Square/1 -> Sum/1
  Square1/1 -> Sum/2
  Square Root/1 -> v_d/1
  Sum/1 -> Square Root/1

== system Switching_06/Unicycle 1/State Feedback Exact Trajectory Controller/Differential Flatness/Subsystem1 ==
  x_dot : Inport
  x_dotdot : Inport  Port=2
  y_dot : Inport  Port=3
  y_dotdot : Inport  Port=4
  Divide : Product  Inputs=*/
  MATLAB Function : MATLAB Function  TreatAsAtomicUnit=on
  Product : Product
  Product1 : Product
  Square : Math  Operator=square
  Square1 : Math  Operator=square
  Sum : Sum  Inputs=+-
  Sum1 : Sum
  w_d : Outport
  wires:
  Product/1 -> Sum/1
  Product1/1 -> Sum/2
  Sum/1 -> Divide/1
  Divide/1 -> w_d/1
  x_dot/1 -> Square/1, Product/1
  y_dotdot/1 -> Product/2
  y_dot/1 -> Product1/2, Square1/1
  MATLAB Function/1(u) -> Divide/2
  Sum1/1 -> MATLAB Function/1("u ")
  Square/1 -> Sum1/1
  Square1/1 -> Sum1/2
  x_dotdot/1 -> Product1/1

== system Switching_06/Unicycle 1/State Feedback Exact Trajectory Controller/Differential Flatness/Subsystem2 ==
  y_dot : Inport
  x_dot : Inport  Port=2
  Atan2 : Trigonometry  Operator=atan2
  Unwrap : dspsigops/Unwrap  tol=pi  InputProcessing=Columns as channels (frame based)  running=off
  theta_d : Outport
  wires:
  Atan2/1 -> Unwrap/1
  y_dot/1 -> Atan2/1
  x_dot/1 -> Atan2/2
  Unwrap/1 -> theta_d/1

== system Switching_06/Unicycle 2/State Feedback Exact Trajectory Controller/Differential Flatness/Subsystem ==
  x_dot : Inport
  y_dot : Inport  Port=2
  Square : Math  Operator=square
  Square Root : Sqrt
  Square1 : Math  Operator=square
  Sum : Sum
  v_d : Outport
  wires:
  x_dot/1 -> Square/1
  y_dot/1 -> Square1/1
  Square/1 -> Sum/1
  Square1/1 -> Sum/2
  Square Root/1 -> v_d/1
  Sum/1 -> Square Root/1

== system Switching_06/Unicycle 2/State Feedback Exact Trajectory Controller/Differential Flatness/Subsystem1 ==
  x_dot : Inport
  x_dotdot : Inport  Port=2
  y_dot : Inport  Port=3
  y_dotdot : Inport  Port=4
  Divide : Product  Inputs=*/
  MATLAB Function : MATLAB Function  TreatAsAtomicUnit=on
  Product : Product
  Product1 : Product
  Square : Math  Operator=square
  Square1 : Math  Operator=square
  Sum : Sum  Inputs=+-
  Sum1 : Sum
  w_d : Outport
  wires:
  Product/1 -> Sum/1
  Product1/1 -> Sum/2
  Sum/1 -> Divide/1
  Divide/1 -> w_d/1
  x_dot/1 -> Square/1, Product/1
  y_dotdot/1 -> Product/2
  y_dot/1 -> Product1/2, Square1/1
  MATLAB Function/1(u) -> Divide/2
  Sum1/1 -> MATLAB Function/1("u ")
  Square/1 -> Sum1/1
  Square1/1 -> Sum1/2
  x_dotdot/1 -> Product1/1

== system Switching_06/Unicycle 2/State Feedback Exact Trajectory Controller/Differential Flatness/Subsystem2 ==
  y_dot : Inport
  x_dot : Inport  Port=2
  Atan2 : Trigonometry  Operator=atan2
  Unwrap : dspsigops/Unwrap  tol=pi  InputProcessing=Columns as channels (frame based)  running=off
  theta_d : Outport
  wires:
  Atan2/1 -> Unwrap/1
  y_dot/1 -> Atan2/1
  x_dot/1 -> Atan2/2
  Unwrap/1 -> theta_d/1

== system Switching_06/Unicycle 3/State Feedback Exact Trajectory Controller/Differential Flatness/Subsystem ==
  x_dot : Inport
  y_dot : Inport  Port=2
  Square : Math  Operator=square
  Square Root : Sqrt
  Square1 : Math  Operator=square
  Sum : Sum
  v_d : Outport
  wires:
  x_dot/1 -> Square/1
  y_dot/1 -> Square1/1
  Square/1 -> Sum/1
  Square1/1 -> Sum/2
  Square Root/1 -> v_d/1
  Sum/1 -> Square Root/1

== system Switching_06/Unicycle 3/State Feedback Exact Trajectory Controller/Differential Flatness/Subsystem1 ==
  x_dot : Inport
  x_dotdot : Inport  Port=2
  y_dot : Inport  Port=3
  y_dotdot : Inport  Port=4
  Divide : Product  Inputs=*/
  MATLAB Function : MATLAB Function  TreatAsAtomicUnit=on
  Product : Product
  Product1 : Product
  Square : Math  Operator=square
  Square1 : Math  Operator=square
  Sum : Sum  Inputs=+-
  Sum1 : Sum
  w_d : Outport
  wires:
  Product/1 -> Sum/1
  Product1/1 -> Sum/2
  Sum/1 -> Divide/1
  Divide/1 -> w_d/1
  x_dot/1 -> Square/1, Product/1
  y_dotdot/1 -> Product/2
  y_dot/1 -> Product1/2, Square1/1
  MATLAB Function/1(u) -> Divide/2
  Sum1/1 -> MATLAB Function/1("u ")
  Square/1 -> Sum1/1
  Square1/1 -> Sum1/2
  x_dotdot/1 -> Product1/1

== system Switching_06/Unicycle 3/State Feedback Exact Trajectory Controller/Differential Flatness/Subsystem2 ==
  y_dot : Inport
  x_dot : Inport  Port=2
  Atan2 : Trigonometry  Operator=atan2
  Unwrap : dspsigops/Unwrap  tol=pi  InputProcessing=Columns as channels (frame based)  running=off
  theta_d : Outport
  wires:
  Atan2/1 -> Unwrap/1
  y_dot/1 -> Atan2/1
  x_dot/1 -> Atan2/2
  Unwrap/1 -> theta_d/1

== matlab function Switching_06/Unicycle 1/State Feedback Exact Trajectory Controller/Differential Flatness/Subsystem1/MATLAB Function ==
  data: u input; u output
function u = fcn(u)

if abs(u)<1e-4
    if u>=0
        u=1e-4;
    else
        u=-1e-4;
    end
else
    u=u;
end

== matlab function Switching_06/Unicycle 2/State Feedback Exact Trajectory Controller/Controller/Transformed Inputs ==
  data: SF_b parameter; SF_xi1 parameter; v_d input; w_d input; e input; u1 output; u2 output
function [u1, u2] = fcn(SF_b, SF_xi1, v_d, w_d, e)

% calculatring values of K
k_1=2*SF_xi1*sqrt(SF_b*v_d+w_d^2);
k_2=SF_b;
k_3=k_1;

% calculating values of u
u1=-k_1*e(1);
u2=-k_2*(v_d*(sin(e(3))/e(3)))*e(2)-k_3*e(3);

== matlab function Switching_06/Unicycle 2/State Feedback Exact Trajectory Controller/Differential Flatness/Subsystem1/MATLAB Function ==
  data: u input; u output
function u = fcn(u)

if abs(u)<1e-4
    if u>=0
        u=1e-4;
    else
        u=-1e-4;
    end
else
    u=u;
end

== matlab function Switching_06/Unicycle 3/State Feedback Exact Trajectory Controller/Controller/MATLAB Function ==
  data: e_w input; e output; theta input
function e  = fcn(e_w, theta)

R=[cos(theta) sin(theta) 0; -sin(theta) cos(theta) 0; 0 0 1];

e=R*e_w;

== matlab function Switching_06/Unicycle 3/State Feedback Exact Trajectory Controller/Controller/Transformed Inputs ==
  data: SF_b parameter; SF_xi1 parameter; v_d input; w_d input; e input; u1 output; u2 output
function [u1, u2] = fcn(SF_b, SF_xi1, v_d, w_d, e)

% calculatring values of K
k_1=2*SF_xi1*sqrt(SF_b*v_d+w_d^2);
k_2=SF_b;
k_3=k_1;

% calculating values of u
u1=-k_1*e(1);
u2=-k_2*(v_d*(sin(e(3))/e(3)))*e(2)-k_3*e(3);

== matlab function Switching_06/Unicycle 3/State Feedback Exact Trajectory Controller/Differential Flatness/Subsystem1/MATLAB Function ==
  data: u input; u output
function u = fcn(u)

if abs(u)<1e-4
    if u>=0
        u=1e-4;
    else
        u=-1e-4;
    end
else
    u=u;
end

== matlab function Switching_06/Unicycle 1/Posture Regulation Controller/MATLAB Function ==
  data: rho input; v output; w output; gamma input; delta input; PR_k1 parameter; PR_k2 parameter; PR_k3 parameter; tolerance_posture parameter
function [v,w] = fcn(rho, gamma, delta, PR_k1, PR_k2, PR_k3, tolerance_posture)

if abs(rho)<tolerance_posture
    v=0;
    w=0;
else
    v=PR_k1*rho*cos(gamma);
    w=PR_k2*gamma+PR_k1*(cos(gamma)*sin(gamma))/gamma*(gamma+PR_k3*delta);
end

== matlab function Switching_06/Unicycle 2/Posture Regulation Controller/MATLAB Function ==
  data: rho input; v output; w output; gamma input; delta input; PR_k1 parameter; PR_k2 parameter; PR_k3 parameter; tolerance_posture parameter
function [v,w] = fcn(rho, gamma, delta, PR_k1, PR_k2, PR_k3, tolerance_posture)

if abs(rho)<tolerance_posture
    v=0;
    w=0;
else
    v=PR_k1*rho*cos(gamma);
    w=PR_k2*gamma+PR_k1*(cos(gamma)*sin(gamma))/gamma*(gamma+PR_k3*delta);
end

== matlab function Switching_06/Unicycle 3/Posture Regulation Controller/MATLAB Function ==
  data: rho input; v output; w output; gamma input; delta input; PR_k1 parameter; PR_k2 parameter; PR_k3 parameter; tolerance_posture parameter
function [v,w] = fcn(rho, gamma, delta, PR_k1, PR_k2, PR_k3, tolerance_posture)

if abs(rho)<tolerance_posture
    v=0;
    w=0;
else
    v=PR_k1*rho*cos(gamma);
    w=PR_k2*gamma+PR_k1*(cos(gamma)*sin(gamma))/gamma*(gamma+PR_k3*delta);
end

== matlab function Switching_06/Unicycle 2/State Feedback Exact Trajectory Controller/Controller/Inverse Transformation ==
  data: v_d input; w_d input; u1 input; v output size=1; u2 input; w output size=1; e input
function [v, w] = fcn(v_d, w_d, u1, u2, e)

v = v_d*cos(e(3))-u1;
w=w_d-u2;

== matlab function Switching_06/Unicycle 2/State Feedback Exact Trajectory Controller/Controller/MATLAB Function ==
  data: e_w input; e output; theta input
function e  = fcn(e_w, theta)

R=[cos(theta) sin(theta) 0; -sin(theta) cos(theta) 0; 0 0 1];

e=R*e_w;

== matlab function Switching_06/Unicycle 3/State Feedback Exact Trajectory Controller/Controller/Inverse Transformation ==
  data: v_d input; w_d input; u1 input; v output size=1; u2 input; w output size=1; e input
function [v, w] = fcn(v_d, w_d, u1, u2, e)

v = v_d*cos(e(3))-u1;
w=w_d-u2;

== matlab function Switching_06/Swittching Logic ==
  data: switching output; v1 input; v2 input; v3 input; w1 input; w2 input; w3 input; switching_out input
function switching = fcn(v1, v2, v3, w1, w2, w3, switching_out)
if switching_out==1
    switching=1;
else
    if v1==0 && v2==0 && v3==0 && w1==0 && w2==0 && w3==0
        switching = 1; 
    else
        switching = 0; 
    end
end

== matlab function Switching_06/Unicycle 1/State Feedback Exact Trajectory Controller/Controller/Inverse Transformation ==
  data: v_d input; w_d input; u1 input; v output size=1; u2 input; w output size=1; e input
function [v, w] = fcn(v_d, w_d, u1, u2, e)

v = v_d*cos(e(3))-u1;
w=w_d-u2;

== matlab function Switching_06/Unicycle 1/State Feedback Exact Trajectory Controller/Controller/MATLAB Function ==
  data: e_w input; e output; theta input
function e  = fcn(e_w, theta)

R=[cos(theta) sin(theta) 0; -sin(theta) cos(theta) 0; 0 0 1];

e=R*e_w;

== matlab function Switching_06/Unicycle 1/State Feedback Exact Trajectory Controller/Controller/Transformed Inputs ==
  data: SF_b parameter; SF_xi1 parameter; v_d input; w_d input; e input; u1 output; u2 output
function [u1, u2] = fcn(SF_b, SF_xi1, v_d, w_d, e)

% calculatring values of K
k_1=2*SF_xi1*sqrt(SF_b*v_d+w_d^2);
k_2=SF_b;
k_3=k_1;

% calculating values of u
u1=-k_1*e(1);
u2=-k_2*(v_d*(sin(e(3))/e(3)))*e(2)-k_3*e(3);
